simulink model "obstacleAvoid_controller"  (R2024b)
settings: configuration reference "obstacleAvoid_controller" (kept outside this file)
undefined symbols (not defined in the file or in its folder): lanes, laneWidth, refSignal, u0
libraries: mpclib x1
settings Model: DataDictionary=obstacleAvoidance_data.sldd  Creator=tshintai  LastModifiedBy=tshintai
settings ConfigSetRef: SourceName=obstacleAvoid_controller

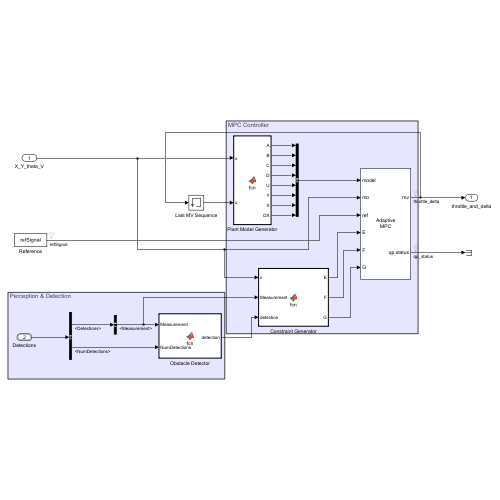
[thumbnail: Simulink's stored preview of the top-level diagram]
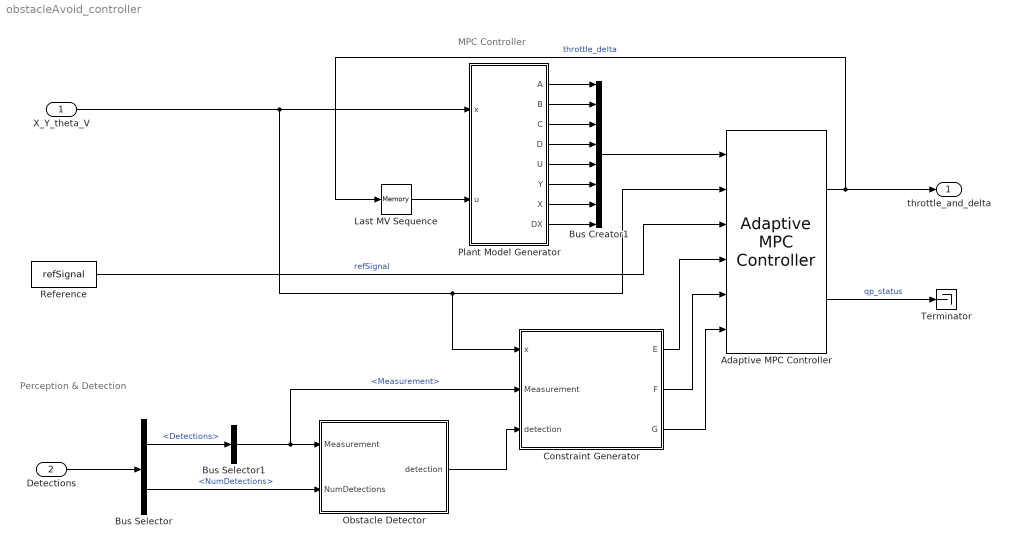
== system obstacleAvoid_controller ==
  note: MPC Controller
  note: Perception & Detection
  X_Y_theta_V : Inport  PortDimensions=4
  Detections : Inport  Port=2  OutDataTypeStr=Bus: BusObjectDetections1
  Adaptive MPC Controller : mpclib/Adaptive MPC Controller  SCDEnableBlockLinearizationSpecification=on  mpcobj=mpcobj  enable_value=0  updateMPCinCallerWorkspace=on  md_inport=off  mv_inport=off  uref_inport=off  return_cost=off  return_mvseq=off  return_qpstatus=on  return_xseq=off  return_state=off  return_ovseq=off  state_inport=off  isltv_plant=off  umin_inport=off  umax_inport=off  ymin_inport=off  ymax_inport=off  cc_inport=on  ywt_inport=off  uwt_inport=off  duwt_inport=off  rhoeps_inport=off  pm_inport=off  MaximumP=10  HorizonChoice=FixedHorizon  BlockDataType=double  SampleTimeInherited=off  switch_inport=off
  Bus Creator1 : BusCreator  Inputs=8
  Bus Selector : BusSelector  OutputSignals=Detections,NumDetections
  Bus Selector1 : BusSelector  OutputSignals=Measurement
  Constraint Generator : MATLAB Function  TreatAsAtomicUnit=on
  Last MV Sequence : Memory  InitialCondition=u0  InheritSampleTime=on
  Obstacle Detector : MATLAB Function  TreatAsAtomicUnit=on
  Plant Model Generator : MATLAB Function  TreatAsAtomicUnit=on
  Reference : Constant  Value=refSignal  VectorParams1D=off
  Terminator : Terminator
  throttle_and_delta : Outport
  wires:
  Bus Selector/1 -> Bus Selector1/1  "<Detections>"
  Obstacle Detector/1(detection) -> Constraint Generator/3(detection)
  Bus Selector1/1 -> Obstacle Detector/1(Measurement), Constraint Generator/2(Measurement)  "<Measurement>"
  Detections/1 -> Bus Selector/1
  Plant Model Generator/7(X) -> Bus Creator1/7
  Adaptive MPC Controller/2 -> Terminator/1  "qp_status"
  Bus Selector/2 -> Obstacle Detector/2(NumDetections)  "<NumDetections>"
  Plant Model Generator/6(Y) -> Bus Creator1/6
  Last MV Sequence/1 -> Plant Model Generator/2(u)
  Bus Creator1/1 -> Adaptive MPC Controller/1
  Plant Model Generator/1(A) -> Bus Creator1/1
  Plant Model Generator/2(B) -> Bus Creator1/2
  X_Y_theta_V/1 -> Adaptive MPC Controller/2, Constraint Generator/1(x), Plant Model Generator/1(x)
  Adaptive MPC Controller/1 -> throttle_and_delta/1, Last MV Sequence/1  "throttle_delta"
  Plant Model Generator/8(DX) -> Bus Creator1/8
  Plant Model Generator/3(C) -> Bus Creator1/3
  Constraint Generator/2(F) -> Adaptive MPC Controller/5
  Constraint Generator/1(E) -> Adaptive MPC Controller/4
  Reference/1 -> Adaptive MPC Controller/3  "refSignal"
  Plant Model Generator/5(U) -> Bus Creator1/5
  Plant Model Generator/4(D) -> Bus Creator1/4
  Constraint Generator/3(G) -> Adaptive MPC Controller/6

== matlab function obstacleAvoid_controller/Obstacle Detector ==
  settings: updateMethod=DISCRETE  sampleTime=TimeStep
  data: Measurement input; NumDetections input; DetectionDistance parameter; detection output
function detection  = fcn(Measurement, NumDetections, DetectionDistance)
% Detection Logic: it determine when the vehicle sees the obstacle
detection = obstacleDetect(Measurement, NumDetections, DetectionDistance);

== matlab function obstacleAvoid_controller/Constraint Generator ==
  settings: updateMethod=DISCRETE  sampleTime=TimeStep
  data: x input; Measurement input; detection input; laneWidth parameter; E output; F output; G output; lanes parameter
function [E,F,G] = fcn(x, Measurement, detection, laneWidth, lanes)
% Generate run-time custom constraint
[E,F,G] = obstacleComputeCustomConstraint(x, Measurement, detection, laneWidth, lanes);

== matlab function obstacleAvoid_controller/Plant Model Generator ==
  settings: updateMethod=DISCRETE  sampleTime=TimeStep
  data: x input; u input; A output; B output; C output; D output; U output size=[2,1]; Y output size=[4,1]; X output size=[4,1]; DX output size=[4,1]; TimeStep parameter
function [A,B,C,D,U,Y,X,DX] = fcn(x,u,TimeStep)
[A,B,C,D,U,Y,X,DX] = obstacleVehicleModelDT(TimeStep,x,u);
